simulink model "wash_out_filter"  (R2021b)
settings: Solver=FixedStepAuto  StartTime=0.0  StopTime=100  FixedStep=0.01  RelTol=1e-3
values from neighbouring files (symbols this model uses):
  Kroll = rollGrad*pi/180    (= 0.0715584993318)    [Init_for_washout_filter.m]
  rx = 0.29    [Init_for_washout_filter.m]    (also in UKF_start.m)
  ry = 0    [Init_for_washout_filter.m]    (also in UKF_start.m)
  T = 0.15    [Init_for_washout_filter.m]
  threshold_vx = 1    [Init_for_washout_filter.m]
settings Model: Creator=thomasperrein  LastModifiedBy=thomasperrein

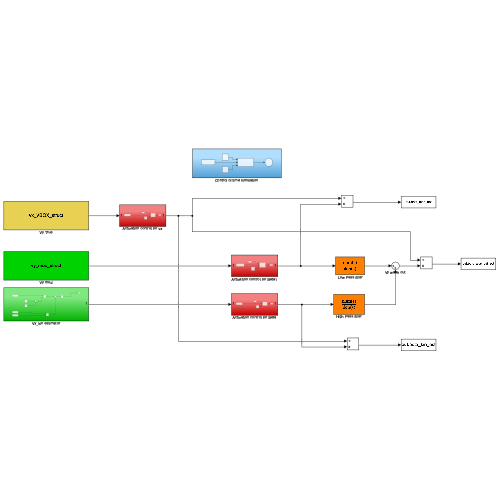
[thumbnail: Simulink's stored preview of the top-level diagram]
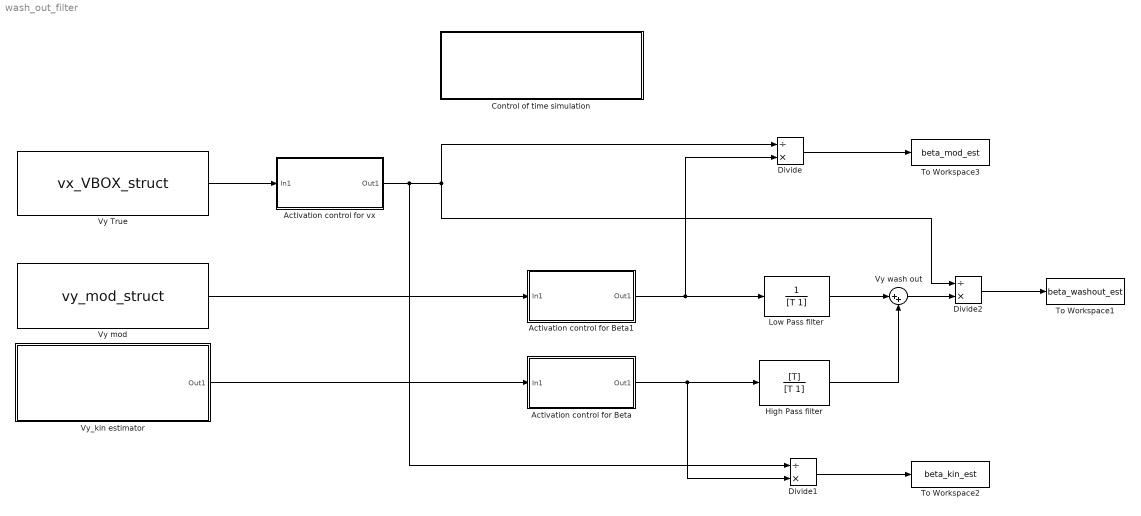
== system wash_out_filter ==
  " Low Pass filter" : TransferFcn  Denominator=[T 1]
  Activation control for Beta : Subsystem
  Activation control for Beta1 : Subsystem
  Activation control for vx : Subsystem
  Control of time simulation : Subsystem
  Divide : Product  Inputs=/*
  Divide1 : Product  Inputs=/*
  Divide2 : Product  Inputs=/*
  High Pass filter : TransferFcn  Numerator=[T]  Denominator=[T 1]
  To Workspace1 : ToWorkspace  VariableName=beta_washout_est  SaveFormat=Timeseries  SampleTime=-1
  To Workspace2 : ToWorkspace  VariableName=beta_kin_est  SaveFormat=Timeseries  SampleTime=-1
  To Workspace3 : ToWorkspace  VariableName=beta_mod_est  SaveFormat=Timeseries  SampleTime=-1
  Vy True : FromWorkspace  VariableName=vx_VBOX_struct
  Vy mod : FromWorkspace  VariableName=vy_mod_struct
  Vy wash out : Sum  Inputs=|++
  Vy_kin estimator : Subsystem
  wires:
  Vy mod/1 -> Activation control for Beta1/1(In1)
  " Low Pass filter"/1 -> Vy wash out/1
  High Pass filter/1 -> Vy wash out/2
  Vy_kin estimator/1(Out1) -> Activation control for Beta/1(In1)
  Activation control for Beta/1(Out1) -> Divide1/2, High Pass filter/1
  Vy wash out/1 -> Divide2/2
  Activation control for Beta1/1(Out1) -> Divide/2, " Low Pass filter"/1
  Vy True/1 -> Activation control for vx/1(In1)
  Divide1/1 -> To Workspace2/1
  Divide/1 -> To Workspace3/1
  Divide2/1 -> To Workspace1/1
  Activation control for vx/1(Out1) -> Divide1/1, Divide2/1, Divide/1

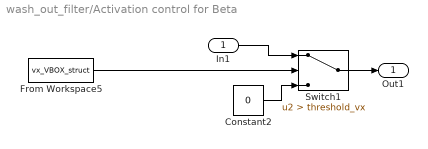
== system wash_out_filter/Activation control for Beta ==
  In1 : Inport
  Constant2 : Constant  Value=0
  From Workspace5 : FromWorkspace  VariableName=vx_VBOX_struct
  Switch1 : Switch  Criteria=u2 > Threshold  Threshold=threshold_vx
  Out1 : Outport
  wires:
  Switch1/1 -> Out1/1
  In1/1 -> Switch1/1
  Constant2/1 -> Switch1/3
  From Workspace5/1 -> Switch1/2

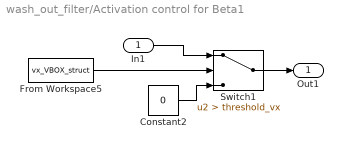
== system wash_out_filter/Activation control for Beta1 ==
  In1 : Inport
  Constant2 : Constant  Value=0
  From Workspace5 : FromWorkspace  VariableName=vx_VBOX_struct
  Switch1 : Switch  Criteria=u2 > Threshold  Threshold=threshold_vx
  Out1 : Outport
  wires:
  Switch1/1 -> Out1/1
  In1/1 -> Switch1/1
  Constant2/1 -> Switch1/3
  From Workspace5/1 -> Switch1/2

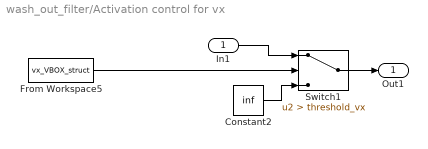
== system wash_out_filter/Activation control for vx ==
  In1 : Inport
  Constant2 : Constant  Value=inf
  From Workspace5 : FromWorkspace  VariableName=vx_VBOX_struct
  Switch1 : Switch  Criteria=u2 > Threshold  Threshold=threshold_vx
  Out1 : Outport
  wires:
  Switch1/1 -> Out1/1
  In1/1 -> Switch1/1
  Constant2/1 -> Switch1/3
  From Workspace5/1 -> Switch1/2

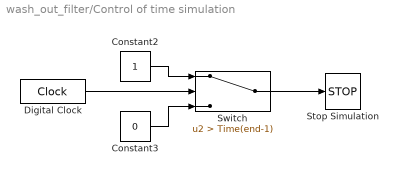
== system wash_out_filter/Control of time simulation ==
  Constant2 : Constant
  Constant3 : Constant  Value=0
  Digital Clock : DigitalClock  SampleTime=0.01
  Stop Simulation : Stop
  Switch : Switch  Criteria=u2 > Threshold  Threshold=Time(end-1)
  wires:
  Constant3/1 -> Switch/3
  Constant2/1 -> Switch/1
  Switch/1 -> Stop Simulation/1
  Digital Clock/1 -> Switch/2

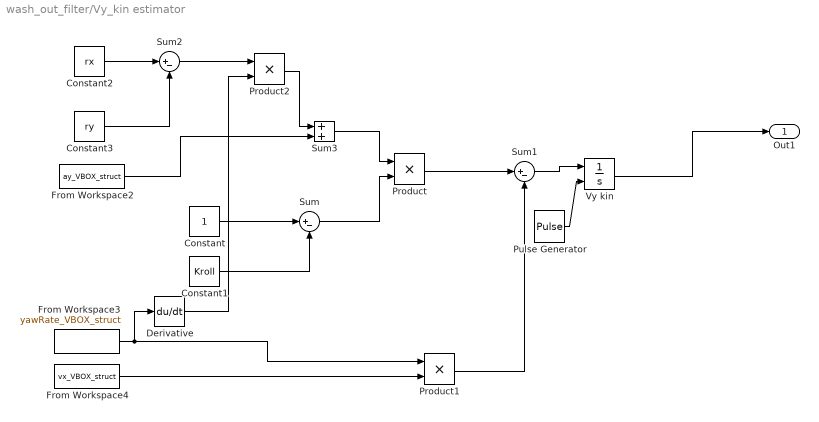
== system wash_out_filter/Vy_kin estimator ==
  Constant : Constant
  Constant1 : Constant  Value=Kroll
  Constant2 : Constant  Value=rx
  Constant3 : Constant  Value=ry
  Derivative : Derivative
  From Workspace2 : FromWorkspace  VariableName=ay_VBOX_struct
  From Workspace3 : FromWorkspace  VariableName=yawRate_VBOX_struct
  From Workspace4 : FromWorkspace  VariableName=vx_VBOX_struct
  Product : Product
  Product1 : Product
  Product2 : Product
  Pulse Generator : DiscretePulseGenerator  PulseType=Time based  Period=4  PulseWidth=5
  Sum : Sum  Inputs=|+-
  Sum1 : Sum  Inputs=|+-
  Sum2 : Sum  Inputs=|+-
  Sum3 : Sum
  Vy kin : Integrator  ExternalReset=rising
  Out1 : Outport
  wires:
  From Workspace3/1 -> Product1/1, Derivative/1
  Constant1/1 -> Sum/2
  Product/1 -> Sum1/1
  Sum/1 -> Product/2
  Constant/1 -> Sum/1
  Product1/1 -> Sum1/2
  Vy kin/1 -> Out1/1
  Sum1/1 -> Vy kin/1
  From Workspace4/1 -> Product1/2
  Constant2/1 -> Sum2/1
  Constant3/1 -> Sum2/2
  Sum2/1 -> Product2/1
  Derivative/1 -> Product2/2
  Product2/1 -> Sum3/1
  From Workspace2/1 -> Sum3/2
  Sum3/1 -> Product/1
  Pulse Generator/1 -> Vy kin/2
